simulink model "ChannelEst_tb"  (R2018b)
settings: Solver=FixedStepAuto  StartTime=1  StopTime=2000  FixedStep=1  RelTol=1e-3
settings Model: PauseTimes=1100  Creator=jason  LastModifiedBy=jason

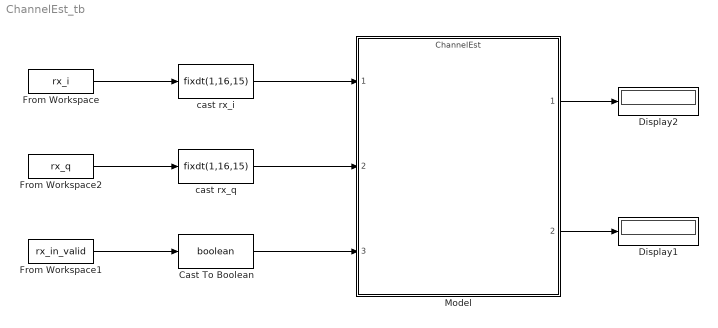
== system ChannelEst_tb ==
  Cast To Boolean : DataTypeConversion  OutDataTypeStr=boolean
  Display1 : Display
  Display2 : Display
  From Workspace : FromWorkspace  VariableName=rx_i  OutDataTypeStr=double  SampleTime=1  Interpolate=off  OutputAfterFinalValue=Setting to zero
  From Workspace1 : FromWorkspace  VariableName=rx_in_valid  OutDataTypeStr=double  SampleTime=1  Interpolate=off  OutputAfterFinalValue=Setting to zero
  From Workspace2 : FromWorkspace  VariableName=rx_q  OutDataTypeStr=double  SampleTime=1  Interpolate=off  OutputAfterFinalValue=Setting to zero
  Model : ModelReference  ModelNameDialog=ChannelEst.slx  SimulationMode=Normal  ModelReferenceVersion=1.46
  cast rx_i : DataTypeConversion  OutDataTypeStr=fixdt(1,16,15)
  cast rx_q : DataTypeConversion  OutDataTypeStr=fixdt(1,16,15)
  wires:
  From Workspace/1 -> cast rx_i/1
  From Workspace2/1 -> cast rx_q/1
  From Workspace1/1 -> Cast To Boolean/1
  cast rx_i/1 -> Model/1
  cast rx_q/1 -> Model/2
  Cast To Boolean/1 -> Model/3
  Model/1 -> Display2/1
  Model/2 -> Display1/1
